simulink model "dg3_Polynomial_masked"  (R2020b)
settings: Solver=ode4  StartTime=0.0  StopTime=6  FixedStep=1e-3  RelTol=1e-3
settings Model: Creator=petir  LastModifiedBy=petir

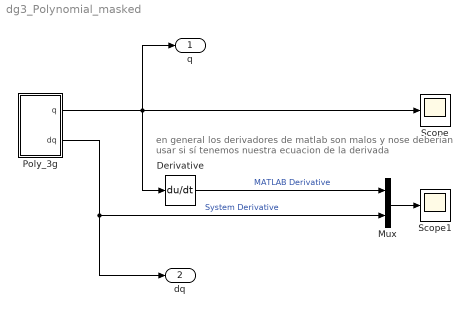
== system dg3_Polynomial_masked ==
  note: en general los derivadores de matlab son malos y nose deberian usar si sí tenemos nuestra ecuacion de la derivada
  Derivative : Derivative
  Mux : Mux  Inputs=2
  Poly_3g : Subsystem  mask{t0=2, tf=5, q0=1, qf=8, v0=-2, vf=0}
      mask prompts: t0 "Tiempo Inicial"; tf "Tiempo Final"; q0 "Posicion inicial"; qf "Pos final"; v0 "Velocidad inicial"; vf "Velocidad final"
      mask init:
      | A = [1 t0 t0^2 t0^3;0 1 2*t0 3*t0^2; 1 tf tf^2 tf^3; 0 1 2*tf 3*tf^2];
      | b = [q0; v0; qf; vf];
      | x = inv(A)*b;
      | a0 = x(1)
      | a1 = x(2)
      | a2 = x(3)
      | a3 = x(4)
  Scope : Scope
  Scope1 : Scope
  q : Outport
  dq : Outport  Port=2
  wires:
  Poly_3g/1(q) -> Scope/1, q/1, Derivative/1
  Poly_3g/2(dq) -> dq/1, Mux/2  "System Derivative"
  Derivative/1 -> Mux/1  "MATLAB Derivative"
  Mux/1 -> Scope1/1

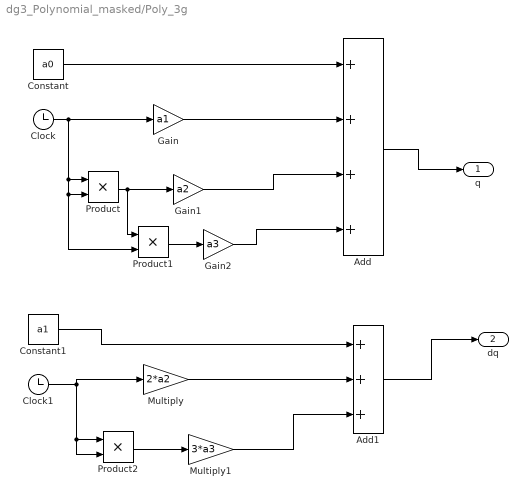
== system dg3_Polynomial_masked/Poly_3g ==
  Add : Sum  Inputs=++++
  Add1 : Sum  Inputs=+++
  Clock : Clock
  Clock1 : Clock
  Constant : Constant  Value=a0
  Constant1 : Constant  Value=a1
  Gain : Gain  Gain=a1
  Gain1 : Gain  Gain=a2
  Gain2 : Gain  Gain=a3
  Multiply : Gain  Gain=2*a2
  Multiply1 : Gain  Gain=3*a3
  Product : Product
  Product1 : Product
  Product2 : Product
  q : Outport
  dq : Outport  Port=2
  wires:
  Gain/1 -> Add/2
  Constant/1 -> Add/1
  Multiply1/1 -> Add1/3
  Add1/1 -> dq/1
  Clock/1 -> Gain/1, Product/1, Product1/2, Product/2
  Product/1 -> Gain1/1, Product1/1
  Constant1/1 -> Add1/1
  Clock1/1 -> Product2/2, Product2/1, Multiply/1
  Multiply/1 -> Add1/2
  Product1/1 -> Gain2/1
  Product2/1 -> Multiply1/1
  Add/1 -> q/1
  Gain1/1 -> Add/3
  Gain2/1 -> Add/4
